simulink model "test01"  (R2025b)
settings: Solver=VariableStepAuto  StartTime=0.0  StopTime=10.0  RelTol=1e-3
settings Model: Creator=sanborkl  LastModifiedBy=sanborkl

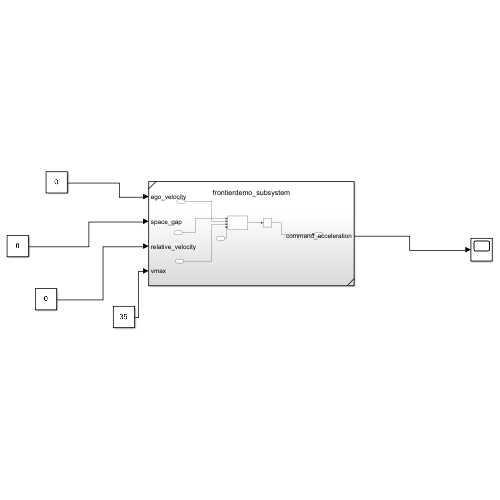
[thumbnail: Simulink's stored preview of the top-level diagram]
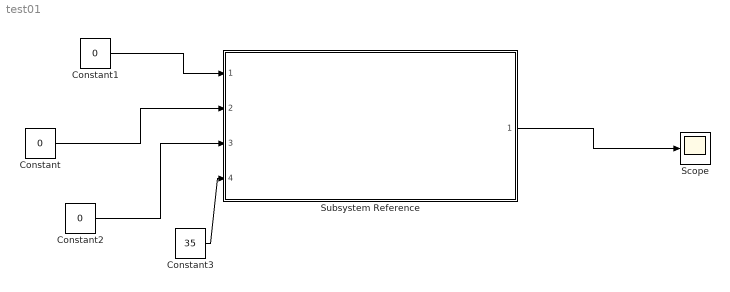
== system test01 ==
  Constant : Constant  Value=0
  Constant1 : Constant  Value=0
  Constant2 : Constant  Value=0
  Constant3 : Constant  Value=35
  Scope : Scope
  Subsystem Reference : Subsystem  ReferencedSubsystem=frontierdemo_subsystem
  wires:
  Constant/1 -> Subsystem Reference/2
  Constant1/1 -> Subsystem Reference/1
  Constant2/1 -> Subsystem Reference/3
  Subsystem Reference/1 -> Scope/1
  Constant3/1 -> Subsystem Reference/4
